simulink model "sist_electrico_prac7_simulink"  (R2025a)
settings: Solver=ode45  StartTime=0.0  StopTime=10.0  RelTol=1e-3
InitFcn:
  | V_a = 24;
  | R = 2;
  | K = 0.01;
  | L = 0.023;
  | J = 0.001;
  | b = 0.0012;
settings Model: Creator=USER  LastModifiedBy=USER

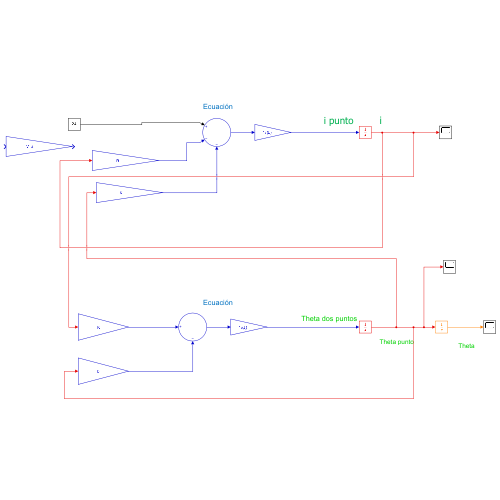
[thumbnail: Simulink's stored preview of the top-level diagram]
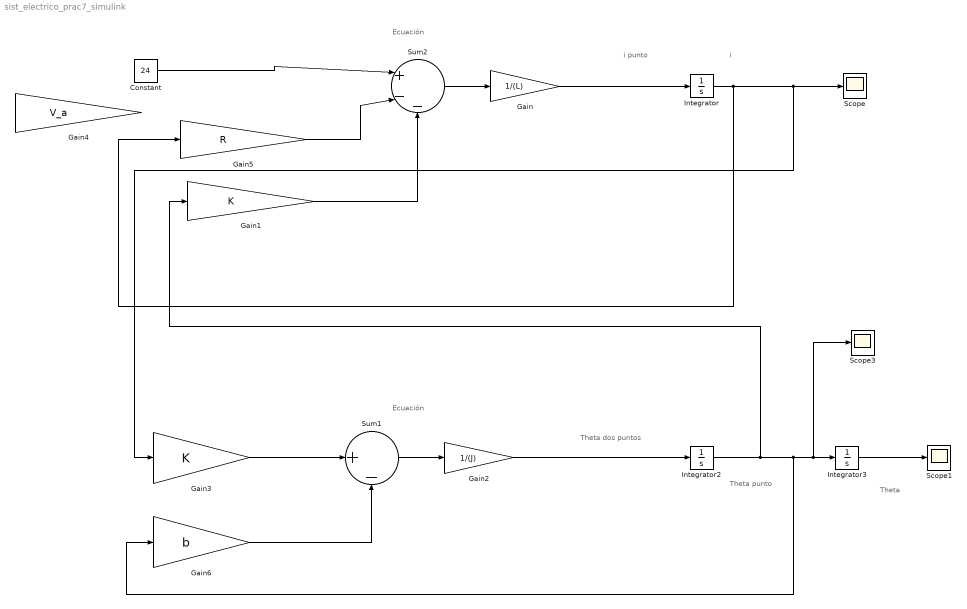
== system sist_electrico_prac7_simulink ==
  note: i
  note: Ecuación
  note: i punto
  note: Theta punto
  note: Ecuación
  note: Theta dos puntos
  note: Theta
  Constant : Constant  Value=24
  Gain : Gain  Gain=1/(L)
  Gain1 : Gain  Gain=K
  Gain2 : Gain  Gain=1/(J)
  Gain3 : Gain  Gain=K
  Gain4 : Gain  Gain=V_a
  Gain5 : Gain  Gain=R
  Gain6 : Gain  Gain=b
  Integrator : Integrator
  Integrator2 : Integrator
  Integrator3 : Integrator
  Scope : Scope
      settings: ActiveDisplayYMinimum=-1.4944101244827284  ActiveDisplayYMaximum=13.449691120344557
  Scope1 : Scope
      settings: ActiveDisplayYMinimum=-110.26755436556266  ActiveDisplayYMaximum=992.40798929006417
  Scope3 : Scope
      settings: ActiveDisplayYMinimum=-12.00013514582438  ActiveDisplayYMaximum=108.00121631241946  DataLoggingVariableName=ScopeData3
  Sum1 : Sum  Inputs=|+-
  Sum2 : Sum  Inputs=|+--
  wires:
  Integrator/1 -> Gain5/1, Scope/1, Gain3/1
  Gain/1 -> Integrator/1
  Integrator3/1 -> Scope1/1
  Integrator2/1 -> Gain6/1, Integrator3/1, Scope3/1, Gain1/1
  Sum2/1 -> Gain/1
  Gain5/1 -> Sum2/2
  Gain1/1 -> Sum2/3
  Gain2/1 -> Integrator2/1
  Sum1/1 -> Gain2/1
  Gain3/1 -> Sum1/1
  Gain6/1 -> Sum1/2
  Constant/1 -> Sum2/1
